simulink model "charges_pneus"  (R2024b)
settings: Solver=VariableStepAuto  StartTime=0.0  StopTime=10.0  RelTol=1e-3
values from neighbouring files (symbols this model uses):
  fr = 0.55    [main_data_vehicle.m]
  g = 9.81    [main_data_vehicle.m]
  h = 0.35    [main_data_vehicle.m]
  L = 1.57    [main_data_vehicle.m]
  m = 240    [main_data_vehicle.m]
settings Model: Creator=marti  LastModifiedBy=marti

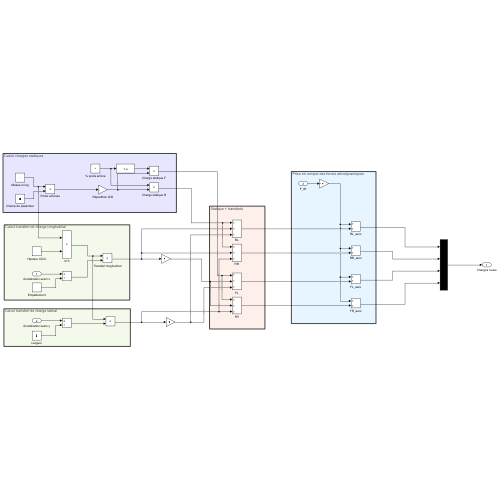
[thumbnail: Simulink's stored preview of the top-level diagram]
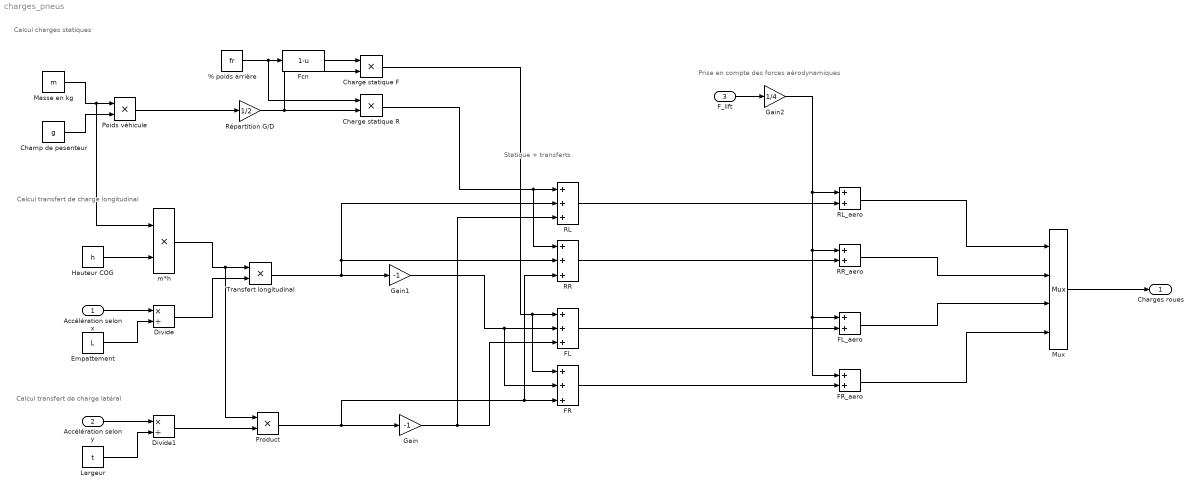
== system charges_pneus ==
  note: Prise en compte des forces aérodynamiques
  note: Statique + transferts
  note: Calcul transfert de charge latéral
  note: Calcul transfert de charge longitudinal
  note: Calcul charges statiques
  Accélération selon x : Inport
  Accélération selon y : Inport  Port=2
  F_lift : Inport  Port=3
  % poids arrière : Constant  Value=fr
  Champ de pesanteur : Constant  Value=g
  Charge statique F : Product
  Charge statique R : Product
  Divide : Product  Inputs=*/
  Divide1 : Product  Inputs=*/
  Empattement : Constant  Value=L
  FL : Sum  Inputs=+++
  FL_aero : Sum
  FR : Sum  Inputs=+++
  FR_aero : Sum
  Fcn : Fcn  Expr=1-u
  Gain : Gain  Gain=-1
  Gain1 : Gain  Gain=-1
  Gain2 : Gain  Gain=1/4
  Hauteur COG : Constant  Value=h
  Largeur : Constant  Value=t
  Masse en kg : Constant  Value=m
  Mux : Mux
  Poids véhicule : Product
  Product : Product
  RL : Sum  Inputs=+++
  RL_aero : Sum
  RR : Sum  Inputs=+++
  RR_aero : Sum
  Répartition G/D : Gain  Gain=1/2
  Transfert longitudinal : Product
  m*h : Product
  Charges roues : Outport
  wires:
  Champ de pesanteur/1 -> Poids véhicule/2
  Masse en kg/1 -> m*h/1, Poids véhicule/1
  Poids véhicule/1 -> Répartition G/D/1
  % poids arrière/1 -> Charge statique R/1, Fcn/1
  Fcn/1 -> Charge statique F/1
  Répartition G/D/1 -> Charge statique F/2, Charge statique R/2
  Hauteur COG/1 -> m*h/2
  Accélération selon x/1 -> Divide/1
  Empattement/1 -> Divide/2
  Divide/1 -> Transfert longitudinal/2
  m*h/1 -> Product/1, Transfert longitudinal/1
  Accélération selon y/1 -> Divide1/1
  Largeur/1 -> Divide1/2
  Divide1/1 -> Product/2
  Product/1 -> RR/3, FR/3, Gain/1
  Gain/1 -> RL/3, FL/3
  Transfert longitudinal/1 -> RR/2, RL/2, Gain1/1
  Gain1/1 -> FR/2, FL/2
  Charge statique F/1 -> FR/1, FL/1
  Charge statique R/1 -> RR/1, RL/1
  RL/1 -> RL_aero/2
  RR/1 -> RR_aero/2
  FL/1 -> FL_aero/2
  FR/1 -> FR_aero/2
  F_lift/1 -> Gain2/1
  Gain2/1 -> FR_aero/1, FL_aero/1, RR_aero/1, RL_aero/1
  RL_aero/1 -> Mux/1
  RR_aero/1 -> Mux/2
  FL_aero/1 -> Mux/3
  FR_aero/1 -> Mux/4
  Mux/1 -> Charges roues/1
